simulink model "e2_p1_model"  (R2020a)
settings: Solver=VariableStepAuto  StartTime=0.0  StopTime=10.0  RelTol=1e-8
undefined symbols (not defined in the file or in its folder): alpha_trim, cD0, cLa, epsilon, g, he, m, rho, S, T_trim, Ve
settings Model: Creator=Tomo  LastModifiedBy=Tomo

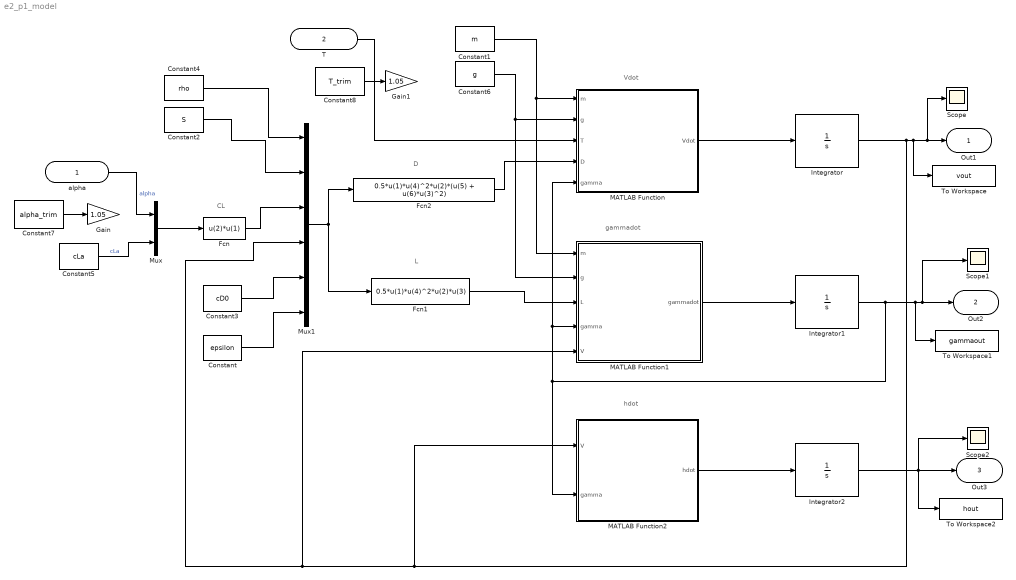
== system e2_p1_model ==
  note: Vdot
  note: D
  note: L
  note: CL
  note: gammadot
  note: hdot
  alpha : Inport
  T : Inport  Port=2
  Constant : Constant  Value=epsilon
  Constant1 : Constant  Value=m
  Constant2 : Constant  Value=S
  Constant3 : Constant  Value=cD0
  Constant4 : Constant  Value=rho
  Constant5 : Constant  Value=cLa
  Constant6 : Constant  Value=g
  Constant7 : Constant  Value=alpha_trim
  Constant8 : Constant  Value=T_trim
  Fcn : Fcn  Expr=u(2)*u(1)
  Fcn1 : Fcn  Expr=0.5*u(1)*u(4)^2*u(2)*u(3)
  Fcn2 : Fcn  Expr=0.5*u(1)*u(4)^2*u(2)*(u(5) + u(6)*u(3)^2)
  Gain : Gain  Gain=1.05
  Gain1 : Gain  Gain=1.05
  Integrator : Integrator  InitialCondition=Ve
  Integrator1 : Integrator
  Integrator2 : Integrator  InitialCondition=he
  MATLAB Function : MATLAB Function  TreatAsAtomicUnit=on
  MATLAB Function1 : MATLAB Function  TreatAsAtomicUnit=on
  MATLAB Function2 : MATLAB Function  TreatAsAtomicUnit=on
  Mux : Mux  Inputs=2
  Mux1 : Mux  Inputs=6
  Scope : Scope
  Scope1 : Scope
  Scope2 : Scope
  To Workspace : ToWorkspace  VariableName=vout  SaveFormat=Structure With Time  SampleTime=-1
  To Workspace1 : ToWorkspace  VariableName=gammaout  SaveFormat=Structure With Time  SampleTime=-1
  To Workspace2 : ToWorkspace  VariableName=hout  SaveFormat=Structure With Time  SampleTime=-1
  Out1 : Outport
  Out2 : Outport  Port=2
  Out3 : Outport  Port=3
  wires:
  Constant5/1 -> Mux/2  "cLa"
  Mux/1 -> Fcn/1
  Constant4/1 -> Mux1/1
  Constant2/1 -> Mux1/2
  Fcn/1 -> Mux1/3
  Constant1/1 -> MATLAB Function1/1(m), MATLAB Function/1(m)
  Constant6/1 -> MATLAB Function1/2(g), MATLAB Function/2(g)
  Mux1/1 -> Fcn1/1, Fcn2/1
  Constant3/1 -> Mux1/5
  Constant/1 -> Mux1/6
  Fcn2/1 -> MATLAB Function/4(D)
  Fcn1/1 -> MATLAB Function1/3(L)
  MATLAB Function/1(Vdot) -> Integrator/1
  MATLAB Function1/1(gammadot) -> Integrator1/1
  MATLAB Function2/1(hdot) -> Integrator2/1
  Integrator1/1 -> MATLAB Function2/2(gamma), MATLAB Function/5(gamma), MATLAB Function1/4(gamma), To Workspace1/1, Scope1/1, Out2/1
  Integrator/1 -> MATLAB Function2/1(V), MATLAB Function1/5(V), Mux1/4, To Workspace/1, Scope/1, Out1/1
  Integrator2/1 -> Scope2/1, Out3/1, To Workspace2/1
  Constant7/1 -> Gain/1
  Constant8/1 -> Gain1/1
  T/1 -> MATLAB Function/3(T)
  alpha/1 -> Mux/1  "alpha"

== matlab function e2_p1_model/MATLAB Function1 ==
  data: m input; gammadot output; g input; L input; gamma input; V input
function gammadot = fcn(m, g, L, gamma, V)
gammadot = (L - m * g * cos(gamma)) / m / V;
end

== matlab function e2_p1_model/MATLAB Function ==
  data: Vdot output; m input; g input; T input; D input; gamma input
function Vdot = fcn(m, g, T, D, gamma)
Vdot = (T - D - m * g * sin(gamma)) / m;
end

== matlab function e2_p1_model/MATLAB Function2 ==
  data: V input; hdot output; gamma input
function hdot = fcn(V, gamma)
hdot = V * sin(gamma);
end
